simulink model "Battery"  (R2023b)
settings: Solver=VariableStepAuto  StartTime=0.0  StopTime=10.0  RelTol=1e-3
libraries: fl_lib x3, nesl_utility x2
settings Model: Creator=user  LastModifiedBy=user

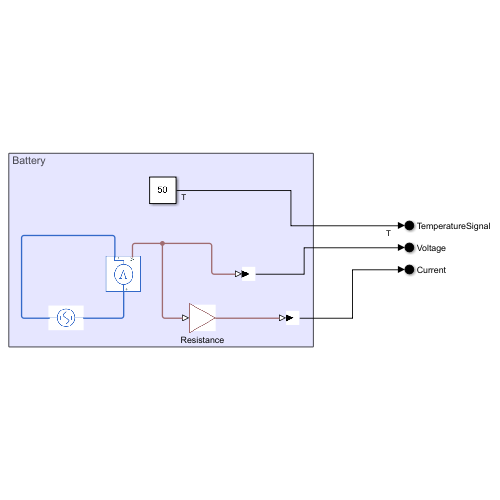
[thumbnail: Simulink's stored preview of the top-level diagram]
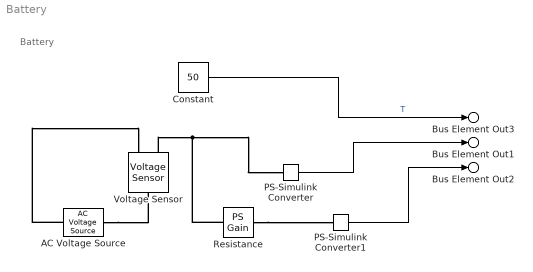
== system Battery ==
  note: Battery
  AC Voltage Source : fl_lib/Electrical/Electrical Sources/AC Voltage Source  amp=1 V  shift=0 deg  frequency=60 Hz  omega=0 rad/s
  Constant : Constant  Value=50
  PS-Simulink Converter : nesl_utility/PS-Simulink Converter  PhysicalDomain=network_engine_domain  SubClassName=ps_output  LeftPortType=input  RightPortType=output  PseudoPeriodic=off  Frequencies=[]  VectorFormat=inherit  Unit=inherit  AffineConversion=off
  PS-Simulink Converter1 : nesl_utility/PS-Simulink Converter  PhysicalDomain=network_engine_domain  SubClassName=ps_output  LeftPortType=input  RightPortType=output  PseudoPeriodic=off  Frequencies=[]  VectorFormat=inherit  Unit=inherit  AffineConversion=off
  Resistance : fl_lib/Physical Signals/Functions/PS Gain  gain=2
  Voltage Sensor : fl_lib/Electrical/Electrical Sensors/Voltage Sensor
  Bus Element Out3 : Outport  PortName=TemperatureSignal
  Bus Element Out1 : Outport  Port=2  PortName=Voltage
  Bus Element Out2 : Outport  Port=3  PortName=Current
  wires:
  PS-Simulink Converter/1 -> Bus Element Out1/1
  PS-Simulink Converter1/1 -> Bus Element Out2/1
  Constant/1 -> Bus Element Out3/1  "T"
  connections:
  Voltage Sensor/RConn1 -- Resistance/LConn1 -- PS-Simulink Converter/LConn1
  AC Voltage Source/LConn1 -- Voltage Sensor/LConn1
  Resistance/RConn1 -- PS-Simulink Converter1/LConn1
  AC Voltage Source/RConn1 -- Voltage Sensor/RConn2
